simulink model "Control_Logic_d"  (R2018b)
settings: Solver=FixedStepAuto  StartTime=Start_time  StopTime=Stop_time  FixedStep=Sample_time  RelTol=1e-3
values from neighbouring files (symbols this model uses):
  Aset_N1 = 2    [Parameter_control.m]
  Aset_N10 = -10    [Parameter_control.m]
  Aset_N11 = 10    [Parameter_control.m]
  Aset_N12 = 20    [Parameter_control.m]
  Aset_N2 = 30    [Parameter_control.m]
  Aset_N3 = 3    [Parameter_control.m]
  Aset_N4 = 5    [Parameter_control.m]
  Aset_N5 = 1    [Parameter_control.m]
  Aset_N6 = 0    [Parameter_control.m]
  Aset_N7 = 0.01    [Parameter_control.m]
  Aset_N8 = 2    [Parameter_control.m]
  Aset_N9 = 0.1    [Parameter_control.m]
  Dset_N1 = 1    [Parameter_control.m]
  Dset_N2 = 1    [Parameter_control.m]
  Sample_time = 0.1    [main.m]    (also in test_tool_initialize.m)
(part 2 of 2)

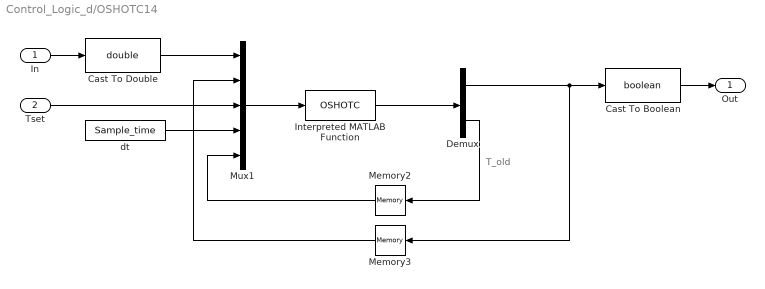
== system Control_Logic_d/OSHOTC14 ==
  note: T_old
  In : Inport
  Tset : Inport  Port=2
  Cast To Boolean : DataTypeConversion  OutDataTypeStr=boolean
  Cast To Double : DataTypeConversion  OutDataTypeStr=double
  Demux : Demux  Outputs=2
  Interpreted MATLAB Function : MATLABFcn  MATLABFcn=OSHOTC
  Memory2 : Memory  InheritSampleTime=on
  Memory3 : Memory  InheritSampleTime=on  LinearizeAsDelay=on
  Mux1 : Mux  Inputs=5
  dt : Constant  Value=Sample_time  OutDataTypeStr=double  SampleTime=Sample_time
  Out : Outport
  wires:
  Cast To Double/1 -> Mux1/1
  In/1 -> Cast To Double/1
  Memory3/1 -> Mux1/2
  Tset/1 -> Mux1/3
  dt/1 -> Mux1/4
  Memory2/1 -> Mux1/5
  Demux/2 -> Memory2/1
  Mux1/1 -> Interpreted MATLAB Function/1
  Cast To Boolean/1 -> Out/1
  Demux/1 -> Cast To Boolean/1, Memory3/1
  Interpreted MATLAB Function/1 -> Demux/1

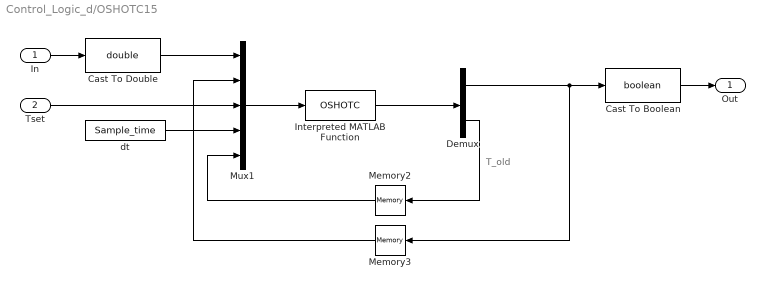
== system Control_Logic_d/OSHOTC15 ==
  note: T_old
  In : Inport
  Tset : Inport  Port=2
  Cast To Boolean : DataTypeConversion  OutDataTypeStr=boolean
  Cast To Double : DataTypeConversion  OutDataTypeStr=double
  Demux : Demux  Outputs=2
  Interpreted MATLAB Function : MATLABFcn  MATLABFcn=OSHOTC
  Memory2 : Memory  InheritSampleTime=on
  Memory3 : Memory  InheritSampleTime=on  LinearizeAsDelay=on
  Mux1 : Mux  Inputs=5
  dt : Constant  Value=Sample_time  OutDataTypeStr=double  SampleTime=Sample_time
  Out : Outport
  wires:
  Interpreted MATLAB Function/1 -> Demux/1
  Demux/1 -> Memory3/1, Cast To Boolean/1
  Cast To Boolean/1 -> Out/1
  Mux1/1 -> Interpreted MATLAB Function/1
  Demux/2 -> Memory2/1
  Memory2/1 -> Mux1/5
  dt/1 -> Mux1/4
  Tset/1 -> Mux1/3
  Memory3/1 -> Mux1/2
  In/1 -> Cast To Double/1
  Cast To Double/1 -> Mux1/1

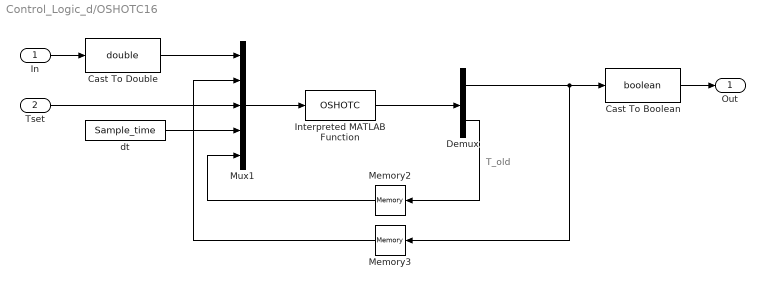
== system Control_Logic_d/OSHOTC16 ==
  note: T_old
  In : Inport
  Tset : Inport  Port=2
  Cast To Boolean : DataTypeConversion  OutDataTypeStr=boolean
  Cast To Double : DataTypeConversion  OutDataTypeStr=double
  Demux : Demux  Outputs=2
  Interpreted MATLAB Function : MATLABFcn  MATLABFcn=OSHOTC
  Memory2 : Memory  InheritSampleTime=on
  Memory3 : Memory  InheritSampleTime=on  LinearizeAsDelay=on
  Mux1 : Mux  Inputs=5
  dt : Constant  Value=Sample_time  OutDataTypeStr=double  SampleTime=Sample_time
  Out : Outport
  wires:
  Interpreted MATLAB Function/1 -> Demux/1
  Demux/1 -> Memory3/1, Cast To Boolean/1
  Cast To Boolean/1 -> Out/1
  Mux1/1 -> Interpreted MATLAB Function/1
  Demux/2 -> Memory2/1
  Memory2/1 -> Mux1/5
  dt/1 -> Mux1/4
  Tset/1 -> Mux1/3
  Memory3/1 -> Mux1/2
  In/1 -> Cast To Double/1
  Cast To Double/1 -> Mux1/1

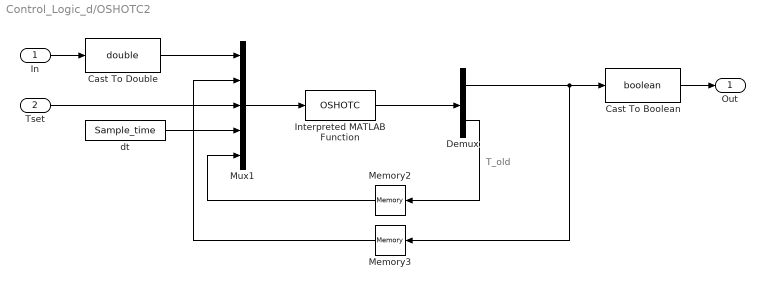
== system Control_Logic_d/OSHOTC2 ==
  note: T_old
  In : Inport
  Tset : Inport  Port=2
  Cast To Boolean : DataTypeConversion  OutDataTypeStr=boolean
  Cast To Double : DataTypeConversion  OutDataTypeStr=double
  Demux : Demux  Outputs=2
  Interpreted MATLAB Function : MATLABFcn  MATLABFcn=OSHOTC
  Memory2 : Memory  InheritSampleTime=on
  Memory3 : Memory  InheritSampleTime=on  LinearizeAsDelay=on
  Mux1 : Mux  Inputs=5
  dt : Constant  Value=Sample_time  OutDataTypeStr=double  SampleTime=Sample_time
  Out : Outport
  wires:
  Cast To Double/1 -> Mux1/1
  In/1 -> Cast To Double/1
  Memory3/1 -> Mux1/2
  Tset/1 -> Mux1/3
  dt/1 -> Mux1/4
  Memory2/1 -> Mux1/5
  Demux/2 -> Memory2/1
  Mux1/1 -> Interpreted MATLAB Function/1
  Cast To Boolean/1 -> Out/1
  Demux/1 -> Cast To Boolean/1, Memory3/1
  Interpreted MATLAB Function/1 -> Demux/1

== system Control_Logic_d/OSHOTC3 ==
  note: T_old
  In : Inport
  Tset : Inport  Port=2
  Cast To Boolean : DataTypeConversion  OutDataTypeStr=boolean
  Cast To Double : DataTypeConversion  OutDataTypeStr=double
  Demux : Demux  Outputs=2
  Interpreted MATLAB Function : MATLABFcn  MATLABFcn=OSHOTC
  Memory2 : Memory  InheritSampleTime=on
  Memory3 : Memory  InheritSampleTime=on  LinearizeAsDelay=on
  Mux1 : Mux  Inputs=5
  dt : Constant  Value=Sample_time  OutDataTypeStr=double  SampleTime=Sample_time
  Out : Outport
  wires:
  Interpreted MATLAB Function/1 -> Demux/1
  Demux/1 -> Memory3/1, Cast To Boolean/1
  Cast To Boolean/1 -> Out/1
  Mux1/1 -> Interpreted MATLAB Function/1
  Demux/2 -> Memory2/1
  Memory2/1 -> Mux1/5
  dt/1 -> Mux1/4
  Tset/1 -> Mux1/3
  Memory3/1 -> Mux1/2
  In/1 -> Cast To Double/1
  Cast To Double/1 -> Mux1/1

== system Control_Logic_d/OSHOTC4 ==
  note: T_old
  In : Inport
  Tset : Inport  Port=2
  Cast To Boolean : DataTypeConversion  OutDataTypeStr=boolean
  Cast To Double : DataTypeConversion  OutDataTypeStr=double
  Demux : Demux  Outputs=2
  Interpreted MATLAB Function : MATLABFcn  MATLABFcn=OSHOTC
  Memory2 : Memory  InheritSampleTime=on
  Memory3 : Memory  InheritSampleTime=on  LinearizeAsDelay=on
  Mux1 : Mux  Inputs=5
  dt : Constant  Value=Sample_time  OutDataTypeStr=double  SampleTime=Sample_time
  Out : Outport
  wires:
  Interpreted MATLAB Function/1 -> Demux/1
  Demux/1 -> Memory3/1, Cast To Boolean/1
  Cast To Boolean/1 -> Out/1
  Mux1/1 -> Interpreted MATLAB Function/1
  Demux/2 -> Memory2/1
  Memory2/1 -> Mux1/5
  dt/1 -> Mux1/4
  Tset/1 -> Mux1/3
  Memory3/1 -> Mux1/2
  In/1 -> Cast To Double/1
  Cast To Double/1 -> Mux1/1

== system Control_Logic_d/OSHOTC5 ==
  note: T_old
  In : Inport
  Tset : Inport  Port=2
  Cast To Boolean : DataTypeConversion  OutDataTypeStr=boolean
  Cast To Double : DataTypeConversion  OutDataTypeStr=double
  Demux : Demux  Outputs=2
  Interpreted MATLAB Function : MATLABFcn  MATLABFcn=OSHOTC
  Memory2 : Memory  InheritSampleTime=on
  Memory3 : Memory  InheritSampleTime=on  LinearizeAsDelay=on
  Mux1 : Mux  Inputs=5
  dt : Constant  Value=Sample_time  OutDataTypeStr=double  SampleTime=Sample_time
  Out : Outport
  wires:
  Cast To Double/1 -> Mux1/1
  In/1 -> Cast To Double/1
  Memory3/1 -> Mux1/2
  Tset/1 -> Mux1/3
  dt/1 -> Mux1/4
  Memory2/1 -> Mux1/5
  Demux/2 -> Memory2/1
  Mux1/1 -> Interpreted MATLAB Function/1
  Cast To Boolean/1 -> Out/1
  Demux/1 -> Cast To Boolean/1, Memory3/1
  Interpreted MATLAB Function/1 -> Demux/1

== system Control_Logic_d/OSHOTC6 ==
  note: T_old
  In : Inport
  Tset : Inport  Port=2
  Cast To Boolean : DataTypeConversion  OutDataTypeStr=boolean
  Cast To Double : DataTypeConversion  OutDataTypeStr=double
  Demux : Demux  Outputs=2
  Interpreted MATLAB Function : MATLABFcn  MATLABFcn=OSHOTC
  Memory2 : Memory  InheritSampleTime=on
  Memory3 : Memory  InheritSampleTime=on  LinearizeAsDelay=on
  Mux1 : Mux  Inputs=5
  dt : Constant  Value=Sample_time  OutDataTypeStr=double  SampleTime=Sample_time
  Out : Outport
  wires:
  Cast To Double/1 -> Mux1/1
  In/1 -> Cast To Double/1
  Memory3/1 -> Mux1/2
  Tset/1 -> Mux1/3
  dt/1 -> Mux1/4
  Memory2/1 -> Mux1/5
  Demux/2 -> Memory2/1
  Mux1/1 -> Interpreted MATLAB Function/1
  Cast To Boolean/1 -> Out/1
  Demux/1 -> Cast To Boolean/1, Memory3/1
  Interpreted MATLAB Function/1 -> Demux/1

== system Control_Logic_d/OSHOTC7 ==
  note: T_old
  In : Inport
  Tset : Inport  Port=2
  Cast To Boolean : DataTypeConversion  OutDataTypeStr=boolean
  Cast To Double : DataTypeConversion  OutDataTypeStr=double
  Demux : Demux  Outputs=2
  Interpreted MATLAB Function : MATLABFcn  MATLABFcn=OSHOTC
  Memory2 : Memory  InheritSampleTime=on
  Memory3 : Memory  InheritSampleTime=on  LinearizeAsDelay=on
  Mux1 : Mux  Inputs=5
  dt : Constant  Value=Sample_time  OutDataTypeStr=double  SampleTime=Sample_time
  Out : Outport
  wires:
  Interpreted MATLAB Function/1 -> Demux/1
  Demux/1 -> Memory3/1, Cast To Boolean/1
  Cast To Boolean/1 -> Out/1
  Mux1/1 -> Interpreted MATLAB Function/1
  Demux/2 -> Memory2/1
  Memory2/1 -> Mux1/5
  dt/1 -> Mux1/4
  Tset/1 -> Mux1/3
  Memory3/1 -> Mux1/2
  In/1 -> Cast To Double/1
  Cast To Double/1 -> Mux1/1

== system Control_Logic_d/OSHOTC8 ==
  note: T_old
  In : Inport
  Tset : Inport  Port=2
  Cast To Boolean : DataTypeConversion  OutDataTypeStr=boolean
  Cast To Double : DataTypeConversion  OutDataTypeStr=double
  Demux : Demux  Outputs=2
  Interpreted MATLAB Function : MATLABFcn  MATLABFcn=OSHOTC
  Memory2 : Memory  InheritSampleTime=on
  Memory3 : Memory  InheritSampleTime=on  LinearizeAsDelay=on
  Mux1 : Mux  Inputs=5
  dt : Constant  Value=Sample_time  OutDataTypeStr=double  SampleTime=Sample_time
  Out : Outport
  wires:
  Cast To Double/1 -> Mux1/1
  In/1 -> Cast To Double/1
  Memory3/1 -> Mux1/2
  Tset/1 -> Mux1/3
  dt/1 -> Mux1/4
  Memory2/1 -> Mux1/5
  Demux/2 -> Memory2/1
  Mux1/1 -> Interpreted MATLAB Function/1
  Cast To Boolean/1 -> Out/1
  Demux/1 -> Cast To Boolean/1, Memory3/1
  Interpreted MATLAB Function/1 -> Demux/1

== system Control_Logic_d/OSHOTC9 ==
  note: T_old
  In : Inport
  Tset : Inport  Port=2
  Cast To Boolean : DataTypeConversion  OutDataTypeStr=boolean
  Cast To Double : DataTypeConversion  OutDataTypeStr=double
  Demux : Demux  Outputs=2
  Interpreted MATLAB Function : MATLABFcn  MATLABFcn=OSHOTC
  Memory2 : Memory  InheritSampleTime=on
  Memory3 : Memory  InheritSampleTime=on  LinearizeAsDelay=on
  Mux1 : Mux  Inputs=5
  dt : Constant  Value=Sample_time  OutDataTypeStr=double  SampleTime=Sample_time
  Out : Outport
  wires:
  Interpreted MATLAB Function/1 -> Demux/1
  Demux/1 -> Memory3/1, Cast To Boolean/1
  Cast To Boolean/1 -> Out/1
  Mux1/1 -> Interpreted MATLAB Function/1
  Demux/2 -> Memory2/1
  Memory2/1 -> Mux1/5
  dt/1 -> Mux1/4
  Tset/1 -> Mux1/3
  Memory3/1 -> Mux1/2
  In/1 -> Cast To Double/1
  Cast To Double/1 -> Mux1/1

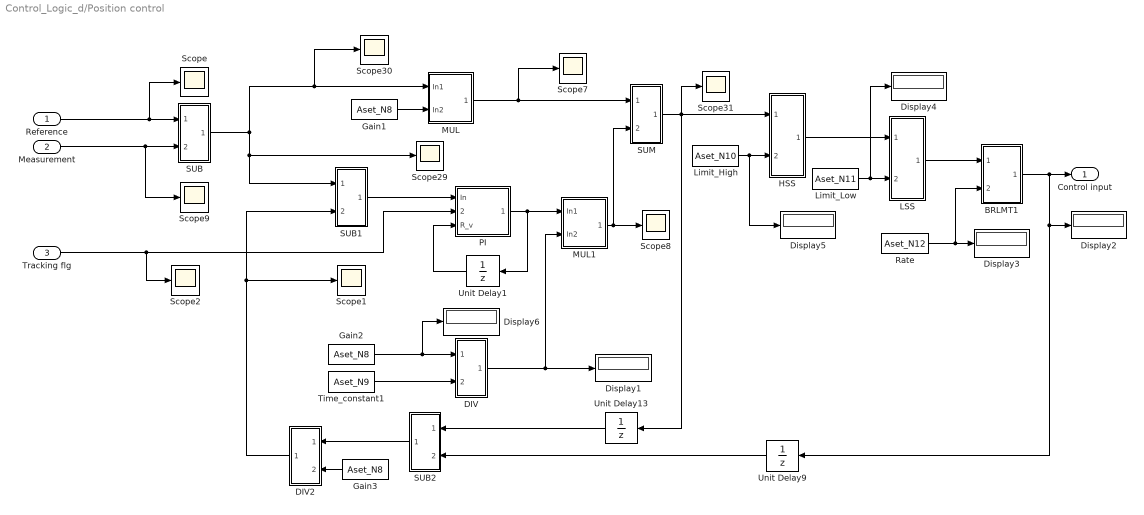
== system Control_Logic_d/Position control ==
  Reference : Inport
  Measurement : Inport  Port=2
  Tracking flg : Inport  Port=3
  BRLMT1 : Subsystem
  DIV : Subsystem
  DIV2 : Subsystem
  Display{1..6} (6 alike) : Display
  Gain1 : Constant  Value=Aset_N8  OutDataTypeStr=double  SampleTime=Sample_time
  Gain2 : Constant  Value=Aset_N8  OutDataTypeStr=double  SampleTime=Sample_time
  Gain3 : Constant  Value=Aset_N8  OutDataTypeStr=double  SampleTime=Sample_time
  HSS : Subsystem
  LSS : Subsystem
  Limit_High : Constant  Value=Aset_N10  OutDataTypeStr=double  SampleTime=Sample_time
  Limit_Low : Constant  Value=Aset_N11  OutDataTypeStr=double  SampleTime=Sample_time
  MUL : Subsystem
  MUL1 : Subsystem
  PI : Subsystem
  Rate : Constant  Value=Aset_N12  OutDataTypeStr=double  SampleTime=Sample_time
  SUB : Subsystem
  SUB1 : Subsystem
  SUB2 : Subsystem
  SUM : Subsystem
  Scope{,1..2,7..9,29..31} (9 alike) : Scope
  Time_constant1 : Constant  Value=Aset_N9  OutDataTypeStr=double  SampleTime=Sample_time
  Unit Delay1 : UnitDelay  SampleTime=Sample_time
  Unit Delay13 : UnitDelay  SampleTime=Sample_time
  Unit Delay9 : UnitDelay  SampleTime=Sample_time
  Control input : Outport
  wires:
  SUM/1(Out) -> Unit Delay13/1, HSS/1(In1), Scope31/1
  Measurement/1 -> Scope9/1, SUB/2(In2)
  SUB/1(Out) -> MUL/1(In1), Scope30/1, SUB1/1(In1), Scope29/1
  Unit Delay13/1 -> SUB2/1(In1)
  MUL/1(Out1) -> SUM/1(In1), Scope7/1
  SUB2/1(Out) -> DIV2/1(In1)
  SUB1/1(Out) -> PI/1(In)
  Gain1/1 -> MUL/2(In2)
  LSS/1(Out1) -> BRLMT1/1(In1)
  Reference/1 -> Scope/1, SUB/1(In1)
  Gain3/1 -> DIV2/2(In2)
  Limit_Low/1 -> Display4/1, LSS/2(In2)
  Tracking flg/1 -> PI/2(Reset), Scope2/1
  PI/1(Out1) -> Unit Delay1/1, MUL1/1(In1)
  Limit_High/1 -> Display5/1, HSS/2(In2)
  MUL1/1(Out1) -> SUM/2(In2), Scope8/1
  BRLMT1/1(Out1) -> Display2/1, Unit Delay9/1, Control input/1
  Time_constant1/1 -> DIV/2(In2)
  Gain2/1 -> Display6/1, DIV/1(In1)
  HSS/1(Out1) -> LSS/1(In1)
  DIV2/1(Out1) -> Scope1/1, SUB1/2(In2)
  Unit Delay9/1 -> SUB2/2(In2)
  DIV/1(Out1) -> Display1/1, MUL1/2(In2)
  Rate/1 -> Display3/1, BRLMT1/2(In2)
  Unit Delay1/1 -> PI/3(R_v)

== system Control_Logic_d/SUB ==
  In1 : Inport
  In2 : Inport  Port=2
  Interpreted MATLAB Function : MATLABFcn  MATLABFcn=SUB
  Mux : Mux  Inputs=2
  Out : Outport
  wires:
  In2/1 -> Mux/2
  Interpreted MATLAB Function/1 -> Out/1
  Mux/1 -> Interpreted MATLAB Function/1
  In1/1 -> Mux/1

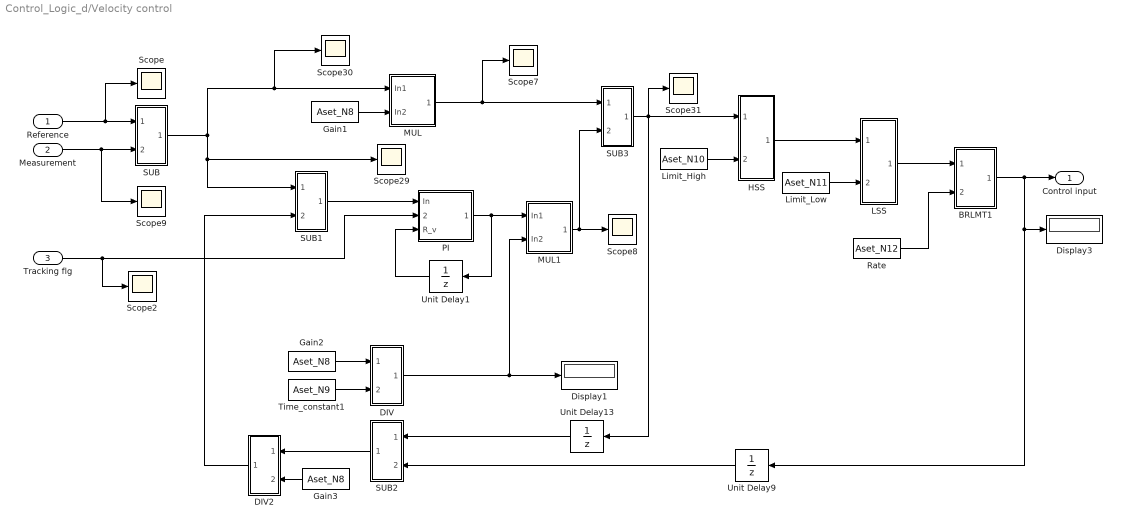
== system Control_Logic_d/Velocity control ==
  Reference : Inport
  Measurement : Inport  Port=2
  Tracking flg : Inport  Port=3
  BRLMT1 : Subsystem
  DIV : Subsystem
  DIV2 : Subsystem
  Display1 : Display
  Display3 : Display
  Gain1 : Constant  Value=Aset_N8  OutDataTypeStr=double  SampleTime=Sample_time
  Gain2 : Constant  Value=Aset_N8  OutDataTypeStr=double  SampleTime=Sample_time
  Gain3 : Constant  Value=Aset_N8  OutDataTypeStr=double  SampleTime=Sample_time
  HSS : Subsystem
  LSS : Subsystem
  Limit_High : Constant  Value=Aset_N10  OutDataTypeStr=double  SampleTime=Sample_time
  Limit_Low : Constant  Value=Aset_N11  OutDataTypeStr=double  SampleTime=Sample_time
  MUL : Subsystem
  MUL1 : Subsystem
  PI : Subsystem
  Rate : Constant  Value=Aset_N12  OutDataTypeStr=double  SampleTime=Sample_time
  SUB : Subsystem
  SUB1 : Subsystem
  SUB2 : Subsystem
  SUB3 : Subsystem
  Scope{,2,7..9,29..31} (8 alike) : Scope
  Time_constant1 : Constant  Value=Aset_N9  OutDataTypeStr=double  SampleTime=Sample_time
  Unit Delay1 : UnitDelay  SampleTime=Sample_time
  Unit Delay13 : UnitDelay  SampleTime=Sample_time
  Unit Delay9 : UnitDelay  SampleTime=Sample_time
  Control input : Outport
  wires:
  Gain1/1 -> MUL/2(In2)
  SUB/1(Out) -> MUL/1(In1), Scope30/1, SUB1/1(In1), Scope29/1
  SUB3/1(Out) -> Unit Delay13/1, HSS/1(In1), Scope31/1
  LSS/1(Out1) -> BRLMT1/1(In1)
  Time_constant1/1 -> DIV/2(In2)
  DIV2/1(Out1) -> SUB1/2(In2)
  DIV/1(Out1) -> Display1/1, MUL1/2(In2)
  Limit_Low/1 -> LSS/2(In2)
  MUL/1(Out1) -> SUB3/1(In1), Scope7/1
  Unit Delay13/1 -> SUB2/1(In1)
  Gain3/1 -> DIV2/2(In2)
  SUB2/1(Out) -> DIV2/1(In1)
  SUB1/1(Out) -> PI/1(In)
  Rate/1 -> BRLMT1/2(In2)
  Reference/1 -> Scope/1, SUB/1(In1)
  Measurement/1 -> Scope9/1, SUB/2(In2)
  Unit Delay9/1 -> SUB2/2(In2)
  Limit_High/1 -> HSS/2(In2)
  Tracking flg/1 -> PI/2(Reset), Scope2/1
  PI/1(Out1) -> Unit Delay1/1, MUL1/1(In1)
  Gain2/1 -> DIV/1(In1)
  Unit Delay1/1 -> PI/3(R_v)
  BRLMT1/1(Out1) -> Control input/1, Display3/1, Unit Delay9/1
  MUL1/1(Out1) -> SUB3/2(In2), Scope8/1
  HSS/1(Out1) -> LSS/1(In1)

== system Control_Logic_d/Position control/BRLMT1 ==
  In1 : Inport
  In2 : Inport  Port=2
  BRLMT : MATLABFcn  MATLABFcn=BRLMT  OutputDimensions=1
  Memory : Memory  InheritSampleTime=on  LinearizeMemory=on  LinearizeAsDelay=on
  Mux1 : Mux
  dt : Constant  Value=Sample_time  OutDataTypeStr=double  SampleTime=Sample_time
  Out1 : Outport
  wires:
  In1/1 -> Mux1/1
  Mux1/1 -> BRLMT/1
  In2/1 -> Mux1/3
  dt/1 -> Mux1/4
  Memory/1 -> Mux1/2
  BRLMT/1 -> Memory/1, Out1/1

== system Control_Logic_d/Position control/DIV ==
  In1 : Inport
  In2 : Inport  Port=2
  DIV : MATLABFcn  MATLABFcn=DIV
  Display : Display
  Display1 : Display
  FlowMax1 : Constant  Value=3.402823e+38  OutDataTypeStr=double  SampleTime=Sample_time
  Mux : Mux  Inputs=3
  Out1 : Outport
  wires:
  In2/1 -> Mux/2, Display1/1
  DIV/1 -> Out1/1
  Mux/1 -> DIV/1
  In1/1 -> Display/1, Mux/1
  FlowMax1/1 -> Mux/3

== system Control_Logic_d/Position control/DIV2 ==
  In1 : Inport
  In2 : Inport  Port=2
  DIV : MATLABFcn  MATLABFcn=DIV
  Display : Display
  Display1 : Display
  FlowMax1 : Constant  Value=3.402823e+38  OutDataTypeStr=double  SampleTime=Sample_time
  Mux : Mux  Inputs=3
  Out1 : Outport
  wires:
  In2/1 -> Mux/2, Display1/1
  DIV/1 -> Out1/1
  Mux/1 -> DIV/1
  In1/1 -> Display/1, Mux/1
  FlowMax1/1 -> Mux/3

== system Control_Logic_d/Position control/HSS ==
  In1 : Inport
  In2 : Inport  Port=2
  HSS : MATLABFcn  MATLABFcn=HSS
  Mux : Mux  Inputs=2
  Out1 : Outport
  wires:
  Mux/1 -> HSS/1
  In1/1 -> Mux/1
  HSS/1 -> Out1/1
  In2/1 -> Mux/2

== system Control_Logic_d/Position control/LSS ==
  In1 : Inport
  In2 : Inport  Port=2
  Interpreted MATLAB Function : MATLABFcn  MATLABFcn=LSS
  Mux : Mux  Inputs=2
  Out1 : Outport
  wires:
  Interpreted MATLAB Function/1 -> Out1/1
  Mux/1 -> Interpreted MATLAB Function/1
  In1/1 -> Mux/1
  In2/1 -> Mux/2

== system Control_Logic_d/Position control/MUL ==
  In1 : Inport
  In2 : Inport  Port=2
  Interpreted MATLAB Function : MATLABFcn  MATLABFcn=MUL
  Mux : Mux  Inputs=2
  Out1 : Outport
  wires:
  Interpreted MATLAB Function/1 -> Out1/1
  In2/1 -> Mux/2
  In1/1 -> Mux/1
  Mux/1 -> Interpreted MATLAB Function/1

== system Control_Logic_d/Position control/MUL1 ==
  In1 : Inport
  In2 : Inport  Port=2
  Interpreted MATLAB Function : MATLABFcn  MATLABFcn=MUL
  Mux : Mux  Inputs=2
  Out1 : Outport
  wires:
  Mux/1 -> Interpreted MATLAB Function/1
  In1/1 -> Mux/1
  In2/1 -> Mux/2
  Interpreted MATLAB Function/1 -> Out1/1

== system Control_Logic_d/Position control/PI ==
  In : Inport
  Reset : Inport  Port=2
  R_v : Inport  Port=3
  Cast To Double : DataTypeConversion  OutDataTypeStr=double
  Interpreted MATLAB Function : MATLABFcn  MATLABFcn=PI
  Memory : Memory  InheritSampleTime=on
  Mux : Mux  Inputs=5
  dt : Constant  Value=Sample_time  OutDataTypeStr=double  SampleTime=Sample_time
  Out1 : Outport
  wires:
  In/1 -> Mux/1
  Reset/1 -> Cast To Double/1
  Interpreted MATLAB Function/1 -> Memory/1, Out1/1
  Mux/1 -> Interpreted MATLAB Function/1
  Memory/1 -> Mux/3
  R_v/1 -> Mux/4
  dt/1 -> Mux/5
  Cast To Double/1 -> Mux/2

== system Control_Logic_d/Position control/SUB ==
  In1 : Inport
  In2 : Inport  Port=2
  Interpreted MATLAB Function : MATLABFcn  MATLABFcn=SUB
  Mux : Mux  Inputs=2
  Out : Outport
  wires:
  In2/1 -> Mux/2
  Interpreted MATLAB Function/1 -> Out/1
  Mux/1 -> Interpreted MATLAB Function/1
  In1/1 -> Mux/1

== system Control_Logic_d/Position control/SUB1 ==
  In1 : Inport
  In2 : Inport  Port=2
  Interpreted MATLAB Function : MATLABFcn  MATLABFcn=SUB
  Mux : Mux  Inputs=2
  Out : Outport
  wires:
  In1/1 -> Mux/1
  Mux/1 -> Interpreted MATLAB Function/1
  Interpreted MATLAB Function/1 -> Out/1
  In2/1 -> Mux/2

== system Control_Logic_d/Position control/SUB2 ==
  In1 : Inport
  In2 : Inport  Port=2
  Interpreted MATLAB Function : MATLABFcn  MATLABFcn=SUB
  Mux : Mux  Inputs=2
  Out : Outport
  wires:
  In1/1 -> Mux/1
  Mux/1 -> Interpreted MATLAB Function/1
  Interpreted MATLAB Function/1 -> Out/1
  In2/1 -> Mux/2

== system Control_Logic_d/Position control/SUM ==
  In1 : Inport
  In2 : Inport  Port=2
  Mux : Mux  Inputs=2
  SUM : MATLABFcn  MATLABFcn=SUM
  Out : Outport
  wires:
  In2/1 -> Mux/2
  SUM/1 -> Out/1
  Mux/1 -> SUM/1
  In1/1 -> Mux/1

== system Control_Logic_d/Velocity control/BRLMT1 ==
  In1 : Inport
  In2 : Inport  Port=2
  BRLMT : MATLABFcn  MATLABFcn=BRLMT  OutputDimensions=1
  Memory : Memory  InheritSampleTime=on  LinearizeMemory=on  LinearizeAsDelay=on
  Mux1 : Mux
  dt : Constant  Value=Sample_time  OutDataTypeStr=double  SampleTime=Sample_time
  Out1 : Outport
  wires:
  In1/1 -> Mux1/1
  Mux1/1 -> BRLMT/1
  In2/1 -> Mux1/3
  dt/1 -> Mux1/4
  Memory/1 -> Mux1/2
  BRLMT/1 -> Memory/1, Out1/1

== system Control_Logic_d/Velocity control/DIV ==
  In1 : Inport
  In2 : Inport  Port=2
  DIV : MATLABFcn  MATLABFcn=DIV
  Display : Display
  Display1 : Display
  FlowMax1 : Constant  Value=3.402823e+38  OutDataTypeStr=double  SampleTime=Sample_time
  Mux : Mux  Inputs=3
  Out1 : Outport
  wires:
  In2/1 -> Mux/2, Display1/1
  DIV/1 -> Out1/1
  Mux/1 -> DIV/1
  In1/1 -> Display/1, Mux/1
  FlowMax1/1 -> Mux/3

== system Control_Logic_d/Velocity control/DIV2 ==
  In1 : Inport
  In2 : Inport  Port=2
  DIV : MATLABFcn  MATLABFcn=DIV
  Display : Display
  Display1 : Display
  FlowMax1 : Constant  Value=3.402823e+38  OutDataTypeStr=double  SampleTime=Sample_time
  Mux : Mux  Inputs=3
  Out1 : Outport
  wires:
  In2/1 -> Mux/2, Display1/1
  DIV/1 -> Out1/1
  Mux/1 -> DIV/1
  In1/1 -> Display/1, Mux/1
  FlowMax1/1 -> Mux/3

== system Control_Logic_d/Velocity control/HSS ==
  In1 : Inport
  In2 : Inport  Port=2
  HSS : MATLABFcn  MATLABFcn=HSS
  Mux : Mux  Inputs=2
  Out1 : Outport
  wires:
  Mux/1 -> HSS/1
  In1/1 -> Mux/1
  HSS/1 -> Out1/1
  In2/1 -> Mux/2

== system Control_Logic_d/Velocity control/LSS ==
  In1 : Inport
  In2 : Inport  Port=2
  Interpreted MATLAB Function : MATLABFcn  MATLABFcn=LSS
  Mux : Mux  Inputs=2
  Out1 : Outport
  wires:
  Interpreted MATLAB Function/1 -> Out1/1
  Mux/1 -> Interpreted MATLAB Function/1
  In1/1 -> Mux/1
  In2/1 -> Mux/2

== system Control_Logic_d/Velocity control/MUL ==
  In1 : Inport
  In2 : Inport  Port=2
  Interpreted MATLAB Function : MATLABFcn  MATLABFcn=MUL
  Mux : Mux  Inputs=2
  Out1 : Outport
  wires:
  Interpreted MATLAB Function/1 -> Out1/1
  In2/1 -> Mux/2
  In1/1 -> Mux/1
  Mux/1 -> Interpreted MATLAB Function/1

== system Control_Logic_d/Velocity control/MUL1 ==
  In1 : Inport
  In2 : Inport  Port=2
  Interpreted MATLAB Function : MATLABFcn  MATLABFcn=MUL
  Mux : Mux  Inputs=2
  Out1 : Outport
  wires:
  Mux/1 -> Interpreted MATLAB Function/1
  In1/1 -> Mux/1
  In2/1 -> Mux/2
  Interpreted MATLAB Function/1 -> Out1/1

== system Control_Logic_d/Velocity control/PI ==
  In : Inport
  Reset : Inport  Port=2
  R_v : Inport  Port=3
  Cast To Double : DataTypeConversion  OutDataTypeStr=double
  Interpreted MATLAB Function : MATLABFcn  MATLABFcn=PI
  Memory : Memory  InheritSampleTime=on
  Mux : Mux  Inputs=5
  dt : Constant  Value=Sample_time  OutDataTypeStr=double  SampleTime=Sample_time
  Out1 : Outport
  wires:
  In/1 -> Mux/1
  Reset/1 -> Cast To Double/1
  Interpreted MATLAB Function/1 -> Memory/1, Out1/1
  Mux/1 -> Interpreted MATLAB Function/1
  Memory/1 -> Mux/3
  R_v/1 -> Mux/4
  dt/1 -> Mux/5
  Cast To Double/1 -> Mux/2

== system Control_Logic_d/Velocity control/SUB ==
  In1 : Inport
  In2 : Inport  Port=2
  Interpreted MATLAB Function : MATLABFcn  MATLABFcn=SUB
  Mux : Mux  Inputs=2
  Out : Outport
  wires:
  In2/1 -> Mux/2
  Interpreted MATLAB Function/1 -> Out/1
  Mux/1 -> Interpreted MATLAB Function/1
  In1/1 -> Mux/1

== system Control_Logic_d/Velocity control/SUB1 ==
  In1 : Inport
  In2 : Inport  Port=2
  Interpreted MATLAB Function : MATLABFcn  MATLABFcn=SUB
  Mux : Mux  Inputs=2
  Out : Outport
  wires:
  In1/1 -> Mux/1
  Mux/1 -> Interpreted MATLAB Function/1
  Interpreted MATLAB Function/1 -> Out/1
  In2/1 -> Mux/2

== system Control_Logic_d/Velocity control/SUB2 ==
  In1 : Inport
  In2 : Inport  Port=2
  Interpreted MATLAB Function : MATLABFcn  MATLABFcn=SUB
  Mux : Mux  Inputs=2
  Out : Outport
  wires:
  In1/1 -> Mux/1
  Mux/1 -> Interpreted MATLAB Function/1
  Interpreted MATLAB Function/1 -> Out/1
  In2/1 -> Mux/2

== system Control_Logic_d/Velocity control/SUB3 ==
  In1 : Inport
  In2 : Inport  Port=2
  Interpreted MATLAB Function : MATLABFcn  MATLABFcn=SUB
  Mux : Mux  Inputs=2
  Out : Outport
  wires:
  In2/1 -> Mux/2
  Interpreted MATLAB Function/1 -> Out/1
  Mux/1 -> Interpreted MATLAB Function/1
  In1/1 -> Mux/1
